simulink model "sim_traj_mpc"  (R2020b)
settings: Solver=VariableStepAuto  StartTime=0.0  StopTime=tsim  RelTol=1e-3
values from neighbouring files (symbols this model uses):
  Nlq_y = Nlq    [get_time_traj_data.m]
  Nlq_z = Nlq    [get_time_traj_data.m]
  ref_y = refs_y{n}    [get_sim_traj_data.m]    (also in get_time_traj_data.m = refStepTrajGen(t_y, Ts_y, 2*Nlq_y); init_sim.m = refStepTrajGen(t_y, Ts_y, 2*Nlq_y); print_plots.m = ref_y(1,1:round(length(ref_y)/2)))
  ref_z = refs_z{n}    [get_sim_traj_data.m]    (also in get_time_traj_data.m = refStepTrajGen(t_z, Ts_z, 2*Nlq_z); init_sim.m = refStepTrajGen(t_z, Ts_z, 2*Nlq_z); print_plots.m = ref_z(1,1:round(length(ref_z)/2)))
  x0 = zeros(1,system_y.nx+system_z.nx+system_phi.nx)    [init_sim.m]
undefined symbols (not defined in the file or in its folder): angle_max, angle_min, arate_max, arate_min, f_max, f_min, g, LQ1_phi, m, mpc_y, tau_max, tau_min, Ts_phi, Ts_y, Ts_z, uavPlanarNonlin, vy_max, vy_min, vz_max, vz_min, y_max, y_min, z_max, z_min
settings Model: Creator=zbouc  LastModifiedBy=zboucek
settings DataIOCC: ReturnWorkspaceOutputs=off
settings DebuggingCC: ArithmeticOperatorsInVariantConditions=warning
settings SFSimCC: SimUseLocalCustomCode=off  CustomCodeUndefinedFunction=UseInterfaceOnly
settings RTWCC: RTWUseLocalCustomCode=off

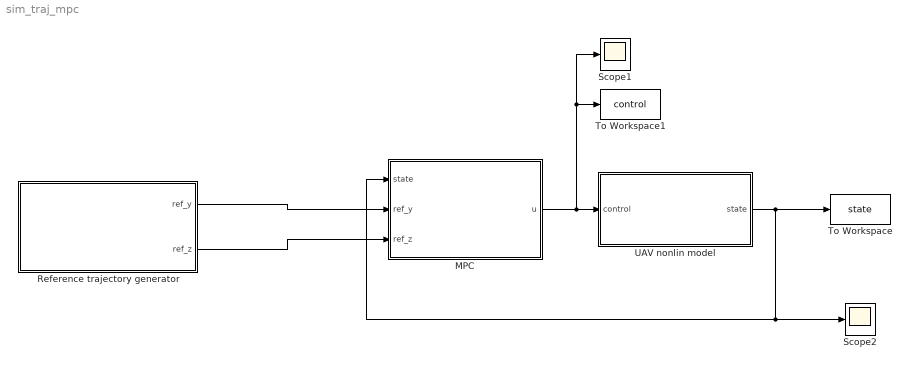
== system sim_traj_mpc ==
  MPC : Subsystem
  Reference trajectory generator : Subsystem
  Scope1 : Scope
  Scope2 : Scope
  To Workspace : ToWorkspace  VariableName=state  SaveFormat=Structure With Time  SampleTime=Ts_phi
  To Workspace1 : ToWorkspace  VariableName=control  SaveFormat=Structure With Time  SampleTime=Ts_phi
  UAV nonlin model : Subsystem
  wires:
  UAV nonlin model/1(state) -> To Workspace/1, Scope2/1, MPC/1(state)
  MPC/1(u) -> UAV nonlin model/1(control), To Workspace1/1, Scope1/1
  Reference trajectory generator/1(ref_y) -> MPC/2(ref_y)
  Reference trajectory generator/2(ref_z) -> MPC/3(ref_z)

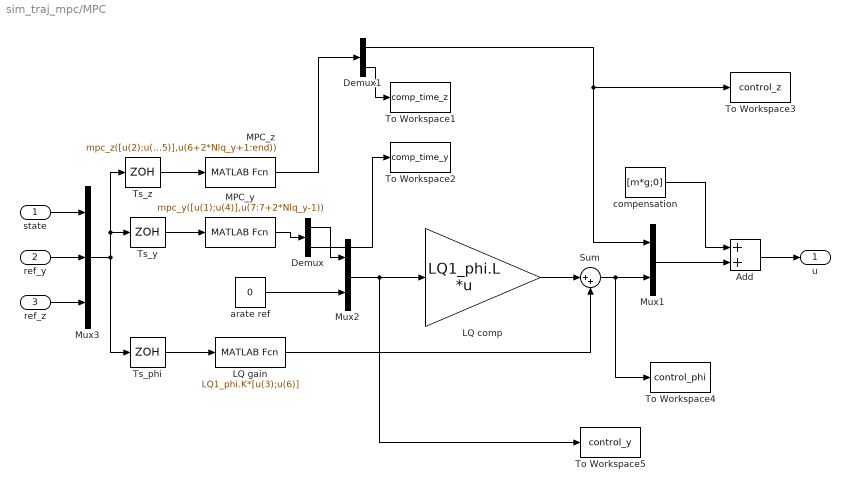
== system sim_traj_mpc/MPC ==
  state : Inport
  ref_y : Inport  Port=2
  ref_z : Inport  Port=3
  Add : Sum
  Demux : Demux  Outputs=2
  Demux1 : Demux  Outputs=2
  LQ comp : Gain  Gain=LQ1_phi.L  Multiplication=Matrix(K*u) (u vector)
  LQ gain : MATLABFcn  MATLABFcn=LQ1_phi.K*[u(3);u(6)]
  MPC_y : MATLABFcn  MATLABFcn=mpc_y([u(1);u(4)],u(7:7+2*Nlq_y-1))
  MPC_z : MATLABFcn  MATLABFcn=mpc_z([u(2);u(5)],u(6+2*Nlq_y+1:end))
  Mux1 : Mux  Inputs=2
  Mux2 : Mux  Inputs=2
  Mux3 : Mux  Inputs=3
  Sum : Sum  Inputs=|++
  To Workspace1 : ToWorkspace  VariableName=comp_time_z  SaveFormat=Structure With Time  SampleTime=Ts_z
  To Workspace2 : ToWorkspace  VariableName=comp_time_y  SaveFormat=Structure With Time  SampleTime=Ts_y
  To Workspace3 : ToWorkspace  VariableName=control_z  SaveFormat=Structure With Time  SampleTime=Ts_z
  To Workspace4 : ToWorkspace  VariableName=control_phi  SaveFormat=Structure With Time  SampleTime=Ts_phi
  To Workspace5 : ToWorkspace  VariableName=control_y  SaveFormat=Structure With Time  SampleTime=Ts_y
  Ts_phi : ZeroOrderHold  SampleTime=Ts_phi
  Ts_y : ZeroOrderHold  SampleTime=Ts_y
  Ts_z : ZeroOrderHold  SampleTime=Ts_z
  arate ref : Constant  Value=0
  compensation : Constant  Value=[m*g;0]
  u : Outport  VectorParamsAs1DForOutWhenUnconnected=off
  wires:
  Mux3/1 -> Ts_phi/1, Ts_z/1, Ts_y/1
  LQ comp/1 -> Sum/1
  Add/1 -> u/1
  Mux1/1 -> Add/2
  Ts_y/1 -> MPC_y/1
  Ts_z/1 -> MPC_z/1
  arate ref/1 -> Mux2/2
  ref_y/1 -> Mux3/2
  state/1 -> Mux3/1
  compensation/1 -> Add/1
  Ts_phi/1 -> LQ gain/1
  LQ gain/1 -> Sum/2
  ref_z/1 -> Mux3/3
  Demux1/2 -> To Workspace1/1
  Demux/2 -> To Workspace2/1
  MPC_y/1 -> Demux/1
  Demux/1 -> Mux2/1
  MPC_z/1 -> Demux1/1
  Demux1/1 -> To Workspace3/1, Mux1/1
  Sum/1 -> To Workspace4/1, Mux1/2
  Mux2/1 -> To Workspace5/1, LQ comp/1

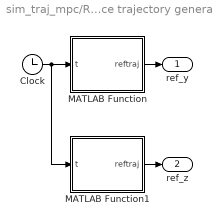
== system sim_traj_mpc/Reference trajectory generator ==
  Clock : Clock
  MATLAB Function : MATLAB Function  TreatAsAtomicUnit=on  SystemSampleTime=Ts_y
  MATLAB Function1 : MATLAB Function  TreatAsAtomicUnit=on  SystemSampleTime=Ts_z
  ref_y : Outport
  ref_z : Outport  Port=2
  wires:
  Clock/1 -> MATLAB Function1/1(t), MATLAB Function/1(t)
  MATLAB Function/1(reftraj) -> ref_y/1
  MATLAB Function1/1(reftraj) -> ref_z/1

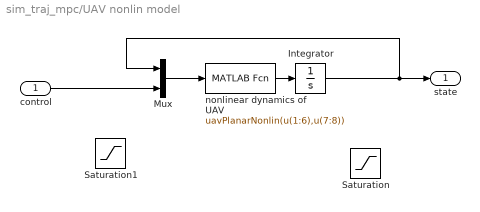
== system sim_traj_mpc/UAV nonlin model ==
  control : Inport
  Integrator : Integrator  InitialCondition=x0
  Mux : Mux  Inputs=2
  Saturation : Saturate  UpperLimit=[y_max;z_max;angle_max;vy_max;vz_max;arate_max]  LowerLimit=[y_min;z_min;angle_min;vy_min;vz_min;arate_min]
  Saturation1 : Saturate  UpperLimit=[f_max; tau_max]  LowerLimit=[f_min; tau_min]
  nonlinear dynamics of UAV : MATLABFcn  MATLABFcn=uavPlanarNonlin(u(1:6),u(7:8))  OutputDimensions=6
  state : Outport  VectorParamsAs1DForOutWhenUnconnected=off
  wires:
  Mux/1 -> nonlinear dynamics of UAV/1
  nonlinear dynamics of UAV/1 -> Integrator/1
  Integrator/1 -> Mux/1, state/1
  control/1 -> Mux/2

== matlab function sim_traj_mpc/Reference trajectory generator/MATLAB Function1 ==
  settings: updateMethod=DISCRETE  sampleTime=Ts_z
  data: t input; reftraj output double size=[2*Nlq_z]; Nlq_z parameter size=1; ref_z parameter; Ts_z parameter
function reftraj = generateTraj_z(t, Nlq_z, ref_z, Ts_z)

k = round(t/Ts_z)+1;
reftraj_temp = reshape(ref_z(:,k:k+Nlq_z-1),[],1);
reftraj = reftraj_temp(1:2*Nlq_z);
end

== matlab function sim_traj_mpc/Reference trajectory generator/MATLAB Function ==
  settings: updateMethod=DISCRETE  sampleTime=Ts_y
  data: t input; reftraj output double size=[2*Nlq_y]; Nlq_y parameter size=1; ref_y parameter; Ts_y parameter size=1
function reftraj = generateTraj_y(t, Nlq_y, ref_y, Ts_y)

k = round(t/Ts_y)+1;
reftraj_temp = reshape(ref_y(:,k:k+Nlq_y-1),[],1);
reftraj = reftraj_temp(1:2*Nlq_y);
end
